simulink model "GNC2026"  (R2024b)
settings: Solver=ode4  StartTime=0.0  StopTime=tsim  FixedStep=baseRate
values from neighbouring files (symbols this model uses):
  a = 1    [Run_Initializer.m]    (also in UKFoptimization.m)
  a1 = 0.236940    (= 0.23694)    [DrawARM.m]    (also in Run_Initializer.m = 2)
  a2 = 0.281536    [DrawARM.m]    (also in Run_Initializer.m = 2)
  a3 = 0.0621    [DrawARM.m]    (also in Run_Initializer.m = 2)
  A_c = eye(3)    [Run_Initializer.m]
  alpha = diag([a1; a2; a3])    [Run_Initializer.m]    (also in overlapping_trajectories.m = alpha_values1(ii); plotTrajectory.m = alpha_values(ii); plotfig.m = alpha_values(ii))
  b = 2    [Run_Initializer.m]    (also in UKFoptimization.m)
  b0 = 0.230400    (= 0.2304)    [DrawARM.m]
  b1 = 0.078980    (= 0.07898)    [DrawARM.m]
  b2 = 0.070384    [DrawARM.m]
  b3 = 0.070685    [DrawARM.m]
  CVrate = 1/5    (= 0.2)    [Run_Initializer.m]
  dt = baseRate    [Run_Initializer.m]    (also in UKFoptimization.m = 0.05; rms_plots.m = median(diff(tA)))
  F_u = zeros(3,1)    [Run_Initializer.m]
  fNum = 1    [Run_Initializer.m]
  gamma = r - (excess + shrink + bracketwidth)    (= 0.05023)    [DrawSpacecraft.m]    (also in Run_Initializer.m = diag([g1; g2; g3]))
  Gamma1_el = 0.12    [Run_Initializer.m]
  Gamma1_sh = 0.005    [Run_Initializer.m]
  Gamma1_wr = 0.025    [Run_Initializer.m]
  Gamma2_el = 5    [Run_Initializer.m]
  Gamma2_sh = 5    [Run_Initializer.m]
  Gamma2_wr = 5    [Run_Initializer.m]
  Gamma3_el = 10    [Run_Initializer.m]
  Gamma3_sh = 40    [Run_Initializer.m]
  Gamma3_wr = 40    [Run_Initializer.m]
  Gamma4_el = 0.039    [Run_Initializer.m]
  Gamma4_sh = 0.015    [Run_Initializer.m]
  Gamma4_wr = 0.029    [Run_Initializer.m]
  Gamma5_el = 800    [Run_Initializer.m]
  Gamma5_sh = 800    [Run_Initializer.m]
  Gamma5_wr = 800    [Run_Initializer.m]
  Gamma6_el = 0.000001    (= 1e-06)    [Run_Initializer.m]
  Gamma6_sh = 0.005    [Run_Initializer.m]
  Gamma6_wr = 0.02    [Run_Initializer.m]
  k = 5    [Run_Initializer.m]    (also in UKFoptimization.m)
  Kd_elarm = 0.8    [Run_Initializer.m]
  Kd_sharm = 1.0    (= 1)    [Run_Initializer.m]
  Kd_wrarm = 0.6    [Run_Initializer.m]
  Kp_elarm = 1.2    [Run_Initializer.m]
  Kp_sharm = 1.5    [Run_Initializer.m]
  Kp_wrarm = 1.0    (= 1)    [Run_Initializer.m]
  Mc_inv = inv(M_c)    [Run_Initializer.m]
  Phi = 73.2749*pi/180    (= 1.27888826407)    [DrawARM.m]
  PWMFreq = 5    [Run_Initializer.m]
  R = [cos(theta) -sin(theta) ... (first row only)    [Run_Initializer.m]    (also in UKFoptimization.m = diag([rx, rx, rt]))
  sep1 = 0.60    (= 0.6)    [Run_Initializer.m]
  sep2 = 0.30    (= 0.3)    [Run_Initializer.m]
  sep3 = 0.30    (= 0.3)    [Run_Initializer.m]
  Tz_lim_elarm = .1    (= 0.1)    [Run_Initializer.m]
  Tz_lim_sharm = .1    (= 0.1)    [Run_Initializer.m]
  Tz_lim_wrarm = .1    (= 0.1)    [Run_Initializer.m]
  VISinLoop = 1    [Run_Initializer.m]
  X1_blk = 0.4    [Run_Initializer.m]
  X2_blk = 0.4    [Run_Initializer.m]
  X3_blk = 0.4    [Run_Initializer.m]
  Y1_blk = 0.4    [Run_Initializer.m]
  Y2_blk = 0.4    [Run_Initializer.m]
  Y3_blk = 0.4    [Run_Initializer.m]
undefined symbols (not defined in the file or in its folder): baseRate, dataRate, DiscIntNeverNeededParam, drop_states_ARM, drop_states_BLACK, drop_states_BLUE, drop_states_RED, F_red_X_nominal, F_red_Y_nominal, F_thrusters_BLACK, F_thrusters_BLUE, F_thrusters_RED, home_states_BLACK, home_states_BLUE, home_states_RED, IBLACK, IBLUE, IDIST, IEE, init_states_BLACK, init_states_BLUE, init_states_RED, IPROX, IRED, K_BLACK, K_BLUE, K_RED, Kd_tb, Kd_tblue, Kd_tr, Kd_xb, Kd_xblue, Kd_xr, Kd_yb, Kd_yblue, Kd_yr, Kp_tb, Kp_tblue, Kp_tr, Kp_xb, Kp_xblue, Kp_xr, Kp_yb, Kp_yblue, Kp_yr, mBLACK, mBLUE, mDIST, mEE, mPROX, mRED, Phase0_End, Phase1_End, Phase2_End, Phase3_End, Phase3_SubPhase1_End, Phase3_SubPhase2_End, Phase3_SubPhase3_End, Phase3_SubPhase4_End, Phase4_End ... (+10)
libraries: simulink x30, nvidiaSharedBlocks x20, MainLibrary x5, dspinverses x3, commrandsrc3 x1, nvidiaIMUSensorslib x1
(part 9 of 9)

== matlab function GNC2026/PhaseSpace Camera Code/Use Hardware to Obtain States/Store BLACK Data/Simulated Noise  (HARDWARE)/Artificial isValid Flag/MATLAB Function1 ==
  data: isValue output; baseRate parameter
function isValue = fcn(baseRate)

persistent k

if isempty(k)
    k = 0;
end

time = k*baseRate;

if time > 65
    isValue = 1;
else
    isValue = 0;
end

k = k+1;

end

== matlab function GNC2026/Navigation Filter/If Action Subsystem/EKF/EKF ==
  data: black_cv_pose input; pose output; velocity output; baseRate parameter; CVrate parameter; confidence output
% Ally Colla
% Chris El-Asmar
% MEKF DOT 2025 

function [pose, velocity, confidence] = MEKF(black_cv_pose, baseRate, CVrate)

persistent converge

if isempty(converge)
    converge = 0;
end

% Different sampling rate
% baseRate = 0.1;

% process noise covariance for propogation
Qx = 1e-8;
Qy = 1e-8;
Qtheta = 1e-8;

% measurement noise covariance for measurement update
Rx = 5e-3;
Ry = 5e-3; 
Rtheta = 5e-3; 
R = diag([Rx, Ry, Rtheta]); 

% filter initial conditions and memory 
persistent x P run theta theta_prev initial_theta
if isempty(run) % check if MEKF has run
    x = zeros(6,1); % x = state vector,(x,y,vx, vy, theta, omega)
    P = diag([1 1 0.05 0.05 1 0.05]); % initial uncertainties based off the spike magnitudes of +/- 1
    run = true;
    theta = 0; 
    theta_prev = 0;
    initial_theta = false;
end

% PROPOGATION

% setting up state transition matrix for 6 dof
phi = eye(6); 
phi(1,3) = baseRate; % updates x position, xnew = x + vx*dt
phi(2,4) = baseRate; % updates y position, ynew = y + vy*dt
phi(5,6) = baseRate; % updates theta position, thetanew = theta + w*dt

x = phi*x; % equation 16 in paper, Wk = 0

% setting up gamma matrix
% take bottom left of matrix in equation 17
% neglecting linear and angular accelerations
% planar rotation only, so no ap (attitude error)
gamma = zeros(6,3);  
gamma(3,1) = 1; % vx
gamma(4,2) = 1; % vy
gamma(6,3) = 1; % omega

Qc = diag([Qx, Qy, Qtheta]);
Qd = Qc*baseRate; % discrete covariance

% calculating covariance of state estimation error
P = phi*P*phi.' + gamma*Qd*gamma.'; 

% MEASUREMENT UPDATE AND OUTLIER REJECTION
yk = black_cv_pose(:); % measurement vector from equation 23

H = zeros(3,6);
H(1,1) = 1; % x
H(2,2) = 1; % y
H(3,5) = 1; % theta

% predicted measurement and innovation
ik = yk - H*x; % innovation equation, before equation 25
if norm(ik) < 0.05
    converge = 1;
end
confidence = converge;

% wrapping theta
wrap = atan2(sin(x(5)), cos(x(5))); % wrap theta from CV
ik(3) = atan2(sin(yk(3) - wrap), cos(yk(3) - wrap)); % wrap the difference

% innovation covariance
E_ik = H*P*H.' + R; % linearized approximation, equation 26 in paper 

% std deviation, expected uncertainty 
sxx = sqrt(max(E_ik(1,1), 1e-10)); % avoids zeros in calculation
syy = sqrt(max(E_ik(2,2), 1e-10));
stt = sqrt(max(E_ik(3,3), 1e-10));

% data falls within 3 std deviations of the mean
k = 3; 

% compare innovation to expected uncertainty 
% flag to see if values are outside 3x std deviation
% values for check become zero if exceeds 3x std dev. 
check_x = abs(ik(1)) <= k * sxx;
check_y = abs(ik(2)) <= k * syy;
check_theta = abs(ik(3)) <= k * stt;

% keep the x,y and theta values that are in the range of 3x std dev.
keep = [check_x; check_y; check_theta];
if any(keep)
    H_new = H(keep, :); % updates H with only the accepted pose
    ik_new = ik(keep); % updates innovation with only the accepted pose
    R_new = diag(diag(R(keep, keep))); % updates covariance matrix and diagonalizes with accepted pose
    Eik_new = H_new*P*H_new.' + R_new; % equation 26 with only accepted pose
    Ks = (P*H_new.')/Eik_new; % kalman gain equation
    x = x + Ks*ik_new; % update states based on kalman gain
    I = eye(6);
    % Joseph form 
    P  = (I - Ks*H_new)*P*(I - Ks*H_new).' + Ks*R_new*Ks.';
end

% keeping theta continuous
if ~initial_theta
    theta_prev = atan2(sin(x(5)), cos(x(5))); % wraps first angle
    theta = theta_prev;
    initial_theta = true;
else
    theta_new = atan2(sin(x(5)), cos(x(5))); 
    true_rotation = atan2(sin(theta_new - theta_prev), ...
                   cos(theta_new - theta_prev)); % wraps the difference for true physical rotation (no 360 jump)
    theta = theta + true_rotation; % previous theta + change in theta wrt time
    theta_prev = theta_new; % set previous theta to new theta to continue loop
end
x(5) = theta; % making theta continuous

% extract positions and velocities from state vector
pose = [x(1); x(2); x(5)];
velocity = [x(3); x(4); x(6)];

end
%%
function [flag] = measurement_flag(baseRate, CVrate)

persistent k
if isempty(k)
    k = 0;
end

flag = 0;

if mod(k,CVrate/baseRate) == 0      
    flag = 1;     % new measurement available
end

k = k + 1;

end

== matlab function GNC2026/Thruster Control Code/Change BLACK Behavior/Rotate Forces to Body/Create Rotation Matrix ==
  data: Rz input; C_bI output
function C_bI = RotateFrame(Rz)

C_bI = [  cos(Rz) sin(Rz)
         -sin(Rz) cos(Rz) ];

end

== matlab function GNC2026/Navigation Filter/If Action Subsystem/UKF/Unscented Kalman Filter ==
  data: x_pre input; x_est output; confidence output; y input; isValid input; P_pre input; P_est output; dt parameter; b parameter; k parameter; a parameter; R parameter; baseRate parameter; CVrate parameter
% Nimish Dhawan
% Sukriti Kumar
% 2025

%%%%%%%%%%%%%%%%%%%%%%%%%%%%%%%%%%%%%%%%%%%%%%%%%%%%%%%%%%%%%%%%%%%%%%%%%
% Inputs
%%%%%%%%%%%%%%%%%%%%%%%%%%%%%%%%%%%%%%%%%%%%%%%%%%%%%%%%%%%%%%%%%%%%%%%%%
% x (6x1)   : state variable [x; y; theta; x_dot; y_dot; theta_dot] 
% X         : Sigma Points
% a, k, b   : unscented transform parameters
% lambda    : scaling parameter
% P (6x6)   : covarience matrix
% S (6x6)   : cholesky decomposition of P

%%%%%%%%%%%%%%%%%%%%%%%%%%%%%%%%%%%%%%%%%%%%%%%%%%%%%%%%%%%%%%%%%%%%%%%%%
% Output
%%%%%%%%%%%%%%%%%%%%%%%%%%%%%%%%%%%%%%%%%%%%%%%%%%%%%%%%%%%%%%%%%%%%%%%%%
% x_est
% P_est

function [x_est, confidence, P_est] = UKF(x_pre, y, isValid, P_pre, dt, b, k, a, R, ...
                                         baseRate, CVrate)

persistent converge

if isempty(converge)
    converge = 0;
end

n = 6;
lambda = a^2 * (n + k) - n;

% Allocating memory
wi_m    = zeros((2*n+1),1);
wi_c    = zeros((2*n+1),1);

% Rotation matrix to go from inertial to relative pose
C3 = eye(3);

% mean and covariance weights (Eq. 4.17f)
for i = 1 : (2*n+1)
    if i == 1
        wi_m(i) = lambda / (n+lambda);
        wi_c(i) = wi_m(i) + 1 - a^2 + b;
    else
        wi_m(i) = 1 / (2 * (n+lambda));
        wi_c(i) = wi_m(i);
    end
end

dynamics = @(x, dt) x + dt * [x(4:6); zeros(3,1)];

% Allocating memory
P_minus = zeros(n,n);
Xi_pre  = zeros(n,(2*n+1));
Fi      = zeros(n,(2*n+1));
x_minus = zeros(n,1);

S_pre = chol(P_pre)';    % Gives lower triangle
Q = 1e-10*eye(n);

% Sigma points calculation 
for i = 1:2*n+1 
    if i == 1
        Xi_pre(:,i) = x_pre;
    elseif i > 1 && i <= n+1
        Xi_pre(:,i) = x_pre + sqrt(n + lambda) * S_pre(:,i-1);
    else
        Xi_pre(:,i) = x_pre - sqrt(n + lambda) * S_pre(:,i-n-1);
    end
end

% Sigma points propagation 
for i = 1 : (2*n+1)
    u = Xi_pre(:,i);
    Fi(:,i) = dynamics(u, dt);
end

% Priori state estimate 
for i = 1 : (2*n+1)
    x_minus = x_minus + wi_m(i) * Fi(:,i);
end

% Priori covariance estimate 
for i = 1 : (2*n+1)
    Pi = wi_c(i) * (Fi(:,i) - x_minus) * (Fi(:,i) - x_minus)' + Q;
    P_minus = P_minus + Pi;
end


% =========================================================================
% CORRECTION
% =========================================================================
Xi_minus = zeros(n,(2*n+1));
h = zeros(3,(2*n+1));    
y_hat = zeros(3,1);     
P_xy = zeros(n,3);
P_yy = zeros(3,3);

S_minus = chol(P_minus)';        % Gives lower triangle

% Sigma points calculation 
for i = 1:2*n+1 
    if i == 1
        Xi_minus(:,i) = x_minus;
    elseif i > 1 && i <= n+1
        Xi_minus(:,i) = x_minus + sqrt(n + lambda) * S_minus(:,i-1);
    else
        Xi_minus(:,i) = x_minus - sqrt(n + lambda) * S_minus(:,i-n-1);
    end
end

% Estimated measurement calculation 
for i = 1 : (2*n+1)
    h(:,i) = C3*Xi_minus(1:3,i);
    y_hat = y_hat + wi_m(i) * h(:,i);
end

% Residual
r = y - y_hat;
if norm(r) < 0.05 % 0.05 works, DO NOT CHANGE (experimentally validated)
    converge = 1;
end
confidence = converge;

% Estimated covariance calculation
for i = 1 : (2*n+1)
    P_yy = P_yy + wi_c(i) * (h(:,i)-y_hat) * (h(:,i)-y_hat)' + R;
    P_xy = P_xy + wi_c(i) * (Xi_minus(:,i) - x_minus) * (h(:,i)-y_hat)';
end

% Posteriori state estimate and covariance 
K = P_xy * inv(P_yy);

P_plus = P_minus - K * P_yy * K';
x_plus = x_minus + K * r;

% Mahalanobis distance

dM          = sqrt(r' * inv(P_yy) * r);
isOutlier   = dM > chi2inv(0.997, 3);

if isOutlier == 1
    P_plus = P_minus;
    x_plus = x_minus;
end

newMeas= measurement_flag(baseRate, CVrate);

if isValid == 1 && newMeas == 1 
    x_est = x_plus;
    P_est = P_plus;
else
    x_est = x_minus;
    P_est = P_minus;
end

end

%%
function [flag] = measurement_flag(baseRate, CVrate)

persistent k
if isempty(k)
    k = 0;
end

flag = 0;

if mod(k,CVrate/baseRate) == 0      
    flag = 1;     % new measurement available
end

k = k + 1;

end

== matlab function GNC2026/Thruster Control Code/Change BLUE Behavior/Calculate Duty Cycle/Generate Initial Guess/MATLAB Function ==
  data: H output; thruster_dist2CG_BLUE parameter; F_thrusters_BLUE parameter
function H = MakeH(thruster_dist2CG_BLUE,F_thrusters_BLUE)

    Vec1 = [ -1
             -1
              0 
              0
              1
              1
              0
              0 ];
          
    Vec2 = [  0
              0
              1
              1
              0
              0
             -1
             -1 ];
         
    Vec3 = thruster_dist2CG_BLUE./1000;
    
    Mat1 = [Vec1, Vec2, Vec3]';
    
    Mat2 = diag((F_thrusters_BLUE./2));
    
    H    = Mat1*Mat2;

end

== matlab function GNC2026/Navigation Filter/If Action Subsystem/EKF/Camera to Inertial Frame ==
  data: r_C_I input; r_T_I output; r_REL_C input
function r_T_I  = CIB(r_C_I, r_REL_C)
l_cam_x    = 0.125; %m, offset in x from origin of Red, left camera
l_cam_y    = 0.03; %m, offset in y from origin of Red, left camera
LAR_x      = 0.145; %m

r_REL_C(1:2) = r_REL_C(1:2) + [l_cam_x; l_cam_y];
th_C         = r_C_I(3);
th_REL       = r_REL_C(3);
th_T         = th_C+th_REL;

C_IC         = [cos(th_C) -sin(th_C); sin(th_C) cos(th_C)]; % Chaser to inertial ref frame rotation matrix
C_IT         = [cos(th_T) -sin(th_T); sin(th_T) cos(th_T)]; % Target to inertial ref frame rotation matrix
xy_T_I       = r_C_I(1:2) + C_IC*r_REL_C(1:2);

r_T_I        = [xy_T_I-C_IT*[LAR_x;0]; th_T];
end

== matlab function GNC2026/Thruster Control Code/Change BLUE Behavior/Calculate Duty Cycle/Rotate Forces to Inertial/Create Rotation Matrix ==
  data: Rz input; C_Ib output
function C_Ib = RotateFrame(Rz)

C_bI = [  cos(Rz) sin(Rz)
         -sin(Rz) cos(Rz) ];

C_Ib = inv(C_bI);

end

== matlab function GNC2026/Simulate Plant Dynamics/BLACK Dynamics/Simulated Noise /Inertial to Camera Frame (SOFTWARE) ==
  data: r_C input; r_REL output; r_T input
% Rotation matrix to go from inertial to relative
function r_REL = CBI(r_C, r_T)
l_cam_x    = 0.125; %m, offset in x from origin of Red, left camera
l_cam_y    = 0.03; %m, offset in y from origin of Red, left camera
th_C       = r_C(3);
th_T       = r_T(3);
d_xy       = r_T(1:2) - r_C(1:2);
C_CI       = [cos(th_C) sin(th_C); -sin(th_C) cos(th_C)]; % Chaser to inertial ref frame rotation matrix
r_REL      = [C_CI*d_xy; th_T - th_C];
r_REL(1:2) = r_REL(1:2) - [l_cam_x; l_cam_y];
end

== matlab function GNC2026/Thruster Control Code/Change BLUE Behavior/Rotate Forces to Body/Create Rotation Matrix ==
  data: Rz input; C_bI output
function C_bI = RotateFrame(Rz)

C_bI = [  cos(Rz) sin(Rz)
         -sin(Rz) cos(Rz) ];

end

== matlab function GNC2026/Thruster Control Code/Change RED Behavior/Calculate Duty Cycle/Generate Initial Guess/MATLAB Function ==
  data: H output; thruster_dist2CG_RED parameter; F_thrusters_RED parameter
function H = MakeH(thruster_dist2CG_RED,F_thrusters_RED)

    Vec1 = [ -1
             -1
              0 
              0
              1
              1
              0
              0 ];
          
    Vec2 = [  0
              0
              1
              1
              0
              0
             -1
             -1 ];
         
    Vec3 = thruster_dist2CG_RED./1000;
    
    Mat1 = [Vec1, Vec2, Vec3]';
    
    Mat2 = diag((F_thrusters_RED./2));
    
    H    = Mat1*Mat2;

end

== matlab function GNC2026/Thruster Control Code/Change RED Behavior/Calculate Duty Cycle/MATLAB Function5 ==
  data: H_final output; u_desired input; duty_cycles output; x0 input; thruster_dist2CG_RED parameter; F_red_X_nominal parameter; F_red_Y_nominal parameter; max_iters parameter; tol parameter
function [H_final, duty_cycles] = optimize_duty_cycle_with_decay( ...
    u_desired, x0, thruster_dist2CG_RED, F_red_X_nominal, F_red_Y_nominal, max_iters, tol)
    %OPTIMIZE_DUTY_CYCLE_WITH_DECAY 
    %   Iteratively optimizes thruster duty cycles while updating thrust decay.
    %
    %   Inputs:
    %       u_desired           - Desired force/torque vector [Fx; Fy; M] (3x1)
    %       x0                  - Initial guess for duty cycles (8x1)
    %       thruster_dist2CG_RED- Distances of thrusters from CG (vector, mm)
    %       F_red_X_nominal     - Nominal X-direction thruster force (scalar, N)
    %       F_red_Y_nominal     - Nominal Y-direction thruster force (scalar, N)
    %       max_iters           - Maximum optimization iterations
    %       tol                 - Convergence tolerance (on duty cycles)
    %
    %   Outputs:
    %       H_final     - Final H-matrix including thrust decay (3x8)
    %       duty_cycles - Optimized duty cycles (8x1)
    %

    % ---------------------------
    % Initialization
    % ---------------------------
    num_thrusters      = length(x0); %#ok<NASGU> % reserved if needed later
    duty_cycles        = x0;                     % current solution
    thrust_decay_factor = 1;                     % initial decay
    prev_duty_cycles   = duty_cycles + 2*tol;    % force first iteration

    % ---------------------------
    % Iterative optimization
    % ---------------------------
    for iter = 1:max_iters
        % Build system matrix H with current decay factor
        H = MakeHWithDecay(thruster_dist2CG_RED, F_red_X_nominal, ...
                           thrust_decay_factor, F_red_Y_nominal);

        % Solve constrained least squares (box constraints: 0 ≤ x ≤ 1)
        duty_cycles = custom_constrained_least_squares(H, u_desired, duty_cycles);

        % Update decay factor based on the current duty cycles
        [thrust_decay_factor, ~] = check_thrust_decay(duty_cycles);

        % Check convergence (∞-norm difference)
        if norm(duty_cycles - prev_duty_cycles, Inf) < tol
            H_final = MakeHWithDecayRecalculateForce(thruster_dist2CG_RED, ...
                        F_red_X_nominal, thrust_decay_factor, F_red_Y_nominal);
            return;
        end

        % Update reference for next iteration
        prev_duty_cycles = duty_cycles;
    end

    % If not converged within max_iters, return final H with last decay
    H_final = MakeHWithDecayRecalculateForce(thruster_dist2CG_RED, ...
                F_red_X_nominal, thrust_decay_factor, F_red_Y_nominal);
end


% ========================================================================
% Custom Constrained Least Squares Solver
% ========================================================================
function x_opt = custom_constrained_least_squares(H, b, x0)
    %CUSTOM_CONSTRAINED_LEAST_SQUARES
    %   Solves min_x ||H*x - b||^2 subject to 0 <= x <= 1
    %   using projected gradient descent with backtracking line search.
    %
    %   Inputs:
    %       H   - System matrix (3x8)
    %       b   - Desired vector (3x1)
    %       x0  - Initial guess (8x1)
    %
    %   Output:
    %       x_opt - Optimal duty cycle vector (8x1)

    % Parameters
    max_iterations = 100;
    tolerance      = 1e-6;
    alpha          = 0.01;  % initial step size
    beta           = 0.5;   % backtracking factor

    % Initialization
    x      = x0;
    x_prev = x0 + 2*tolerance;

    % Precompute matrices
    HtH = H' * H;
    Htb = H' * b;

    for iter = 1:max_iterations
        % Gradient of ||H*x - b||^2
        gradient = 2 * (HtH*x - Htb);

        % Store objective for comparison
        current_obj = norm(H*x - b)^2;

        % Backtracking line search
        step_size = alpha;
        for ls_iter = 1:20
            x_new = x - step_size * gradient;
            x_new = max(0, min(1, x_new)); % project into [0,1]

            new_obj = norm(H*x_new - b)^2;
            if new_obj < current_obj
                break; % accept step
            else
                step_size = step_size * beta;
            end
        end

        % Update
        x = x_new;

        % Convergence check
        if norm(x - x_prev) < tolerance
            break;
        end

        % Adaptive step size tuning
        if iter > 1 && new_obj < current_obj
            alpha = min(alpha * 1.1, 0.1); % speed up if progress
        else
            alpha = alpha * 0.9;           % slow down otherwise
        end

        % Store for next iteration
        x_prev = x;
    end

    x_opt = x;
end


% ========================================================================
% Construct H-matrix (with decay factor)
% ========================================================================
function H = MakeHWithDecay(thruster_dist2CG, F_X_nominal, thrust_decay_factor, F_Y_nominal)
    %MAKEHWITHDECAY
    %   Builds the H matrix that maps thruster duty cycles to [Fx; Fy; M],
    %   applying thrust decay.
    %
    %   Outputs H as (3x8)

    % Convert thruster arm distances to meters
    adjusted_dist = thruster_dist2CG / 1000;

    % Thruster directions (X, Y, and moment arm)
    Vec1 = [-1; -1;  0;  0;  1;  1;  0;  0]; % X
    Vec2 = [ 0;  0;  1;  1;  0;  0; -1; -1]; % Y
    Vec3 = adjusted_dist;                    % moment (Z)

    Mat1 = [Vec1, Vec2, Vec3]';

    % Thruster forces (scaled by decay)
    F_thrusters = [F_X_nominal; F_X_nominal; ...
                   F_Y_nominal; F_Y_nominal; ...
                   F_X_nominal; F_X_nominal; ...
                   F_Y_nominal; F_Y_nominal] * thrust_decay_factor;

    % Build diagonal scaling
    Mat2 = diag(F_thrusters / 2);

    % Final mapping
    H = Mat1 * Mat2;
end


% ========================================================================
% Construct H-matrix (recalculate full force with decay)
% ========================================================================
function H = MakeHWithDecayRecalculateForce(thruster_dist2CG, F_X_nominal, thrust_decay_factor, F_Y_nominal)
    %MAKEHWITHDECAYRECALCULATEFORCE
    %   Same as MakeHWithDecay but applies full nominal force scaling.

    adjusted_dist = thruster_dist2CG / 1000;

    Vec1 = [-1; -1;  0;  0;  1;  1;  0;  0];
    Vec2 = [ 0;  0;  1;  1;  0;  0; -1; -1];
    Vec3 = adjusted_dist;

    Mat1 = [Vec1, Vec2, Vec3]';

    F_thrusters = [F_X_nominal; F_X_nominal; ...
                   F_Y_nominal; F_Y_nominal; ...
                   F_X_nominal; F_X_nominal; ...
                   F_Y_nominal; F_Y_nominal] * thrust_decay_factor;

    Mat2 = diag(F_thrusters);

    H = Mat1 * Mat2;
end


% ========================================================================
% Thrust Decay Update Rule
% ========================================================================
function [thrust_decay_factor, count] = check_thrust_decay(PWMs)
    %CHECK_THRUST_DECAY
    %   Updates thrust decay factor based on average duty cycle.
    %
    %   Inputs:
    %       PWMs - Duty cycle vector (8x1)
    %
    %   Outputs:
    %       thrust_decay_factor - Adjusted decay factor (scalar)
    %       count               - Number of active thrusters

    % Normalize if needed
    if max(PWMs) > 1
        PWMs = PWMs / max(PWMs);
    end
    
    % Active thrusters
    count = sum(PWMs > 0);
    
    % Mean duty cycle (only active thrusters)
    avg_duty = sum(max(PWMs, 0)) / max(count, 1);
    
    % Update rule (piecewise)
    if avg_duty < 0.3 || count == 0
        thrust_decay_factor = 1;
    else
        thrust_decay_factor = max(0.6 - 2*avg_duty + 1, 0.5);
    end
end

== matlab function GNC2026/Thruster Control Code/Change BLUE Behavior/Calculate Duty Cycle/MATLAB Function1 ==
  data: ThrustPer_Final output; ThrustPer input; PWMFreq parameter
function ThrustPer_Final  = ThrusterSat(ThrustPer, PWMFreq)

    ValveTime       = 0.007;
    TControl        = 1/PWMFreq;

    ThrustPer_Final = zeros(8,1);
    
    if max(ThrustPer) > 1
        ThrustPer_Sat = ThrustPer/max(ThrustPer);
    else
        ThrustPer_Sat = ThrustPer;
    end
    
    for i = 1:8
        if ThrustPer_Sat(i) > ValveTime/TControl 
            ThrustPer_Final(i) = ThrustPer_Sat(i);
        else
            ThrustPer_Final(i) = 0;
        end
    end


end

== matlab function GNC2026/Navigation Filter/If Action Subsystem/UKF/Camera to Inertial Frame ==
  data: r_C_I input; r_T_I output; r_REL_C input
function r_T_I  = CIB(r_C_I, r_REL_C)
l_cam_x    = 0.125; %m, offset in x from origin of Red, left camera
l_cam_y    = 0.03;  %m, offset in y from origin of Red, left camera
LAR_x      = 0.145; %m

r_REL_C(1:2) = r_REL_C(1:2) + [l_cam_x; l_cam_y];
th_C         = r_C_I(3);
th_REL       = r_REL_C(3);
th_T         = th_C+th_REL;

C_IC         = [cos(th_C) -sin(th_C); sin(th_C) cos(th_C)]; % Chaser to inertial ref frame rotation matrix
C_IT         = [cos(th_T) -sin(th_T); sin(th_T) cos(th_T)]; % Target to inertial ref frame rotation matrix
xy_T_I       = r_C_I(1:2) + C_IC*r_REL_C(1:2);

r_T_I        = [xy_T_I-C_IT*[LAR_x;0]; th_T];
end

== matlab function GNC2026/Simulate Plant Dynamics/BLACK Dynamics/Simulated Noise /Unwrap/Unwrap/MATLAB Function ==
  data: u input; y output; u_pre input; y_pre input; u_next output
function [y, u_next] = fcn(u, u_pre, y_pre)

% Nimish Dhawan 2025
% Carleton University

%%%%%%%%%%%%%%%%%%%%%%%%%%%%%%%%%%%%%%%%%%%%%%%%%%%%%%%%%%%%%%%%%%%%%%%%%
% Inputs
%%%%%%%%%%%%%%%%%%%%%%%%%%%%%%%%%%%%%%%%%%%%%%%%%%%%%%%%%%%%%%%%%%%%%%%%%
% u (rad)       : current wrapped angle
% u_pre (rad)   : previous wrapped angle
% y_pre (rad)   : previous unwrapped angle

%%%%%%%%%%%%%%%%%%%%%%%%%%%%%%%%%%%%%%%%%%%%%%%%%%%%%%%%%%%%%%%%%%%%%%%%%
% Output
%%%%%%%%%%%%%%%%%%%%%%%%%%%%%%%%%%%%%%%%%%%%%%%%%%%%%%%%%%%%%%%%%%%%%%%%%
% y (rad)       : unwrapped angle
% u_next (rad)  : next wrapped angle

x = mod((u-u_pre)+pi, 2*pi) - pi;

y = y_pre + x;
u_next = u;

end

== matlab function GNC2026/Thruster Control Code/Change RED Behavior/Calculate Duty Cycle/Rotate Forces to Inertial/Create Rotation Matrix ==
  data: Rz input; C_Ib output
function C_Ib = RotateFrame(Rz)

C_bI = [  cos(Rz) sin(Rz)
         -sin(Rz) cos(Rz) ];

C_Ib = inv(C_bI);

end

== matlab function GNC2026/Thruster Control Code/Change RED Behavior/Rotate Forces to Body/Create Rotation Matrix ==
  data: Rz input; C_bI output
function C_bI = RotateFrame(Rz)

C_bI = [  cos(Rz) sin(Rz)
         -sin(Rz) cos(Rz) ];

end

== matlab function GNC2026/Simulate Plant Dynamics/BLACK Dynamics/Simulated Noise /Unwrap/Unwrap1/MATLAB Function ==
  data: u input; y output; y_pre input; init_states_BLACK parameter
function y  = fcn(u, y_pre, init_states_BLACK)

% Nimish Dhawan 2025
% Carleton University

persistent hold

if isempty(hold)
    hold = init_states_BLACK(3);
end

%%%%%%%%%%%%%%%%%%%%%%%%%%%%%%%%%%%%%%%%%%%%%%%%%%%%%%%%%%%%%%%%%%%%%%%%%
% Inputs
%%%%%%%%%%%%%%%%%%%%%%%%%%%%%%%%%%%%%%%%%%%%%%%%%%%%%%%%%%%%%%%%%%%%%%%%%
% u (rad)       : current wrapped angle
% u_pre (rad)   : previous wrapped angle
% y_pre (rad)   : previous unwrapped angle

%%%%%%%%%%%%%%%%%%%%%%%%%%%%%%%%%%%%%%%%%%%%%%%%%%%%%%%%%%%%%%%%%%%%%%%%%
% Output
%%%%%%%%%%%%%%%%%%%%%%%%%%%%%%%%%%%%%%%%%%%%%%%%%%%%%%%%%%%%%%%%%%%%%%%%%
% y (rad)       : unwrapped angle
% u_next (rad)  : next wrapped angle

x = mod((u-hold)+pi, 2*pi) - pi;

y = y_pre + x;
hold = u;

end

== matlab function GNC2026/Navigation Filter/If Action Subsystem/UKF/Unwrap/Unwrap/MATLAB Function ==
  data: u input; y output; u_pre input; y_pre input; u_next output
function [y, u_next] = fcn(u, u_pre, y_pre)

% Nimish Dhawan 2025
% Carleton University

%%%%%%%%%%%%%%%%%%%%%%%%%%%%%%%%%%%%%%%%%%%%%%%%%%%%%%%%%%%%%%%%%%%%%%%%%
% Inputs
%%%%%%%%%%%%%%%%%%%%%%%%%%%%%%%%%%%%%%%%%%%%%%%%%%%%%%%%%%%%%%%%%%%%%%%%%
% u (rad)       : current wrapped angle
% u_pre (rad)   : previous wrapped angle
% y_pre (rad)   : previous unwrapped angle

%%%%%%%%%%%%%%%%%%%%%%%%%%%%%%%%%%%%%%%%%%%%%%%%%%%%%%%%%%%%%%%%%%%%%%%%%
% Output
%%%%%%%%%%%%%%%%%%%%%%%%%%%%%%%%%%%%%%%%%%%%%%%%%%%%%%%%%%%%%%%%%%%%%%%%%
% y (rad)       : unwrapped angle
% u_next (rad)  : next wrapped angle

x = mod((u-u_pre)+pi, 2*pi) - pi;

y = y_pre + x;
u_next = u;

end

== matlab function GNC2026/Navigation Filter/If Action Subsystem/UKF/Unwrap/Unwrap1/MATLAB Function ==
  data: u input; y output; y_pre input; init_states_BLACK parameter
function y  = fcn(u, y_pre, init_states_BLACK)

% Nimish Dhawan 2025
% Carleton University

persistent hold

if isempty(hold)
    hold = init_states_BLACK(3);
end

%%%%%%%%%%%%%%%%%%%%%%%%%%%%%%%%%%%%%%%%%%%%%%%%%%%%%%%%%%%%%%%%%%%%%%%%%
% Inputs
%%%%%%%%%%%%%%%%%%%%%%%%%%%%%%%%%%%%%%%%%%%%%%%%%%%%%%%%%%%%%%%%%%%%%%%%%
% u (rad)       : current wrapped angle
% u_pre (rad)   : previous wrapped angle
% y_pre (rad)   : previous unwrapped angle

%%%%%%%%%%%%%%%%%%%%%%%%%%%%%%%%%%%%%%%%%%%%%%%%%%%%%%%%%%%%%%%%%%%%%%%%%
% Output
%%%%%%%%%%%%%%%%%%%%%%%%%%%%%%%%%%%%%%%%%%%%%%%%%%%%%%%%%%%%%%%%%%%%%%%%%
% y (rad)       : unwrapped angle
% u_next (rad)  : next wrapped angle

x = mod((u-hold)+pi, 2*pi) - pi;

y = y_pre + x;
hold = u;

end

== matlab function GNC2026/Thruster Control Code/Change BLACK Behavior/Calculate Duty Cycle/MATLAB Function1 ==
  data: ThrustPer_Final output; ThrustPer input; PWMFreq parameter
function ThrustPer_Final  = ThrusterSat(ThrustPer, PWMFreq)

    ValveTime       = 0.007;
    TControl        = 1/PWMFreq;

    ThrustPer_Final = zeros(8,1);
    
    if max(ThrustPer) > 1
        ThrustPer_Sat = ThrustPer/max(ThrustPer);
    else
        ThrustPer_Sat = ThrustPer;
    end
    
    for i = 1:8
        if ThrustPer_Sat(i) > ValveTime/TControl 
            ThrustPer_Final(i) = ThrustPer_Sat(i);
        else
            ThrustPer_Final(i) = 0;
        end
    end


end

== matlab function GNC2026/PhaseSpace Camera Code/Use Hardware to Obtain States/Store BLACK Data/Simulated Noise  (HARDWARE)/Sample and Hold ==
  data: y output; u input; CVrate parameter; baseRate parameter
function y  = fcn(u, CVrate, baseRate)
% Description:
% Sampling and holding values
% Input: 
% u [3x1]: CV Data
% Output:
% y [3x1]: Sampled Data

persistent k y_hold

% Initialize 
if isempty(k)
    k = 0;
    y_hold = u;
end

% Sample the value at every second step
if mod(k,CVrate/baseRate) == 0
    y_hold = u;   
end

y = y_hold;

k = k+1;

end

== matlab function GNC2026/3 - Control/Default LQR Control (RED)/Calculate Error/MATLAB Function ==
  data: Rz_path input; Rz_error output; Rz_measured input
function Rz_error = SmoothAngularDifference(Rz_path, Rz_measured)

    Rz_error = mod(Rz_measured-Rz_path+pi, 2*pi)-pi;


end

== matlab function GNC2026/PhaseSpace Camera Code/Use Hardware to Obtain States/Store BLACK Data/Simulated Noise  (HARDWARE)/Unwrap/Unwrap/MATLAB Function ==
  data: u input; y output; u_pre input; y_pre input; u_next output
function [y, u_next] = fcn(u, u_pre, y_pre)

% Nimish Dhawan 2025
% Carleton University

%%%%%%%%%%%%%%%%%%%%%%%%%%%%%%%%%%%%%%%%%%%%%%%%%%%%%%%%%%%%%%%%%%%%%%%%%
% Inputs
%%%%%%%%%%%%%%%%%%%%%%%%%%%%%%%%%%%%%%%%%%%%%%%%%%%%%%%%%%%%%%%%%%%%%%%%%
% u (rad)       : current wrapped angle
% u_pre (rad)   : previous wrapped angle
% y_pre (rad)   : previous unwrapped angle

%%%%%%%%%%%%%%%%%%%%%%%%%%%%%%%%%%%%%%%%%%%%%%%%%%%%%%%%%%%%%%%%%%%%%%%%%
% Output
%%%%%%%%%%%%%%%%%%%%%%%%%%%%%%%%%%%%%%%%%%%%%%%%%%%%%%%%%%%%%%%%%%%%%%%%%
% y (rad)       : unwrapped angle
% u_next (rad)  : next wrapped angle

x = mod((u-u_pre)+pi, 2*pi) - pi;

y = y_pre + x;
u_next = u;

end

== matlab function GNC2026/Simulate Plant Dynamics/BLACK Dynamics/Simulated Noise /Sample and Hold ==
  data: y output; u input; CVrate parameter; baseRate parameter
function y  = fcn(u, CVrate, baseRate)
% Description:
% Sampling and holding values
% Input: 
% u [3x1]: CV Data
% Output:
% y [3x1]: Sampled Data

persistent k y_hold

% Initialize 
if isempty(k)
    k = 0;
    y_hold = u;
end

% Sample the value at every second step
if mod(k,CVrate/baseRate) == 0
    y_hold = u;   
end

y = y_hold;

k = k+1;

end

== matlab function GNC2026/Simulate Plant Dynamics/BLACK Dynamics/Simulated Noise /MATLAB Function1 ==
  data: data output; LARstates_C_B input; isValid output; baseRate parameter
function [data, isValid] = fcn(LARstates_C_B, baseRate)

persistent k

if isempty(k)
    k = 0;
end

time = k*baseRate;

% Extracting LAR states
x = LARstates_C_B(1);
y = LARstates_C_B(2);

% Angle between normal and LOS vector
lambda = atand(y/x);

% Send isValue = 0 when target LAR is out of FOV
% if abs(lambda) > 40
%     isValid = 0;
% else
%     isValid = 1;
% end
isValid = 1;

k = k+1;

if isValid == 1
    data = [0;0;0];
else
    data = LARstates_C_B;
end

% data = LARstates_C_B;
% isValid = 1;

end

== matlab function GNC2026/2 - Guidance/Custom PPL (RED)/End Effector Desired ==
  data: r_C input; r_T_I input; EEdesired output; thRel output; LOS_angle output
function [EEdesired, thRel, LOS_angle] = fcn(r_C, r_T_I)

LARstates_I = r_T_I;

LAR_x = 0.145; % LAR offset in target BoF, m
th_T  = r_T_I(3);
C_IT  = [cos(th_T) -sin(th_T); sin(th_T) cos(th_T)]; % Target to inertial ref frame rotation matrix

LARstates_I(1:2) = r_T_I(1:2) + C_IT*[LAR_x;0];
LARstates_REL = CBI(r_C, LARstates_I);

EEdesired = LARstates_REL + [0.02; 0.15; 0];
thRel     = LARstates_REL(3);
LOS_angle = atan(LARstates_REL(2)/LARstates_REL(1));

end
%%
% Rotation matrix to go from inertial to relative
function r_REL = CBI(r_C, r_T)
th_C       = r_C(3);
th_T       = r_T(3);
d_xy       = r_T(1:2) - r_C(1:2);
C_CI       = [cos(th_C) sin(th_C); -sin(th_C) cos(th_C)]; % Chaser to inertial ref frame rotation matrix
r_REL      = [C_CI*d_xy; th_T - th_C];
r_REL(1:2) = r_REL(1:2);
end

== matlab function GNC2026/Simulate Plant Dynamics/BLACK Dynamics/Simulated Noise /BLK CoM to LAR ==
  data: r_T_I input; LARstates_I output
% Calculates position vector of LAR based on position vector of Target CoM 
function LARstates_I = fcn(r_T_I)

LARstates_I = r_T_I;

LAR_x = 0.145; % LAR offset in target BoF, m
th_T  = r_T_I(3);
C_IT  = [cos(th_T) -sin(th_T); sin(th_T) cos(th_T)]; % Target to inertial ref frame rotation matrix


LARstates_I(1:2) = r_T_I(1:2) + C_IT*[LAR_x;0];

end

== matlab function GNC2026/PhaseSpace Camera Code/Use Hardware to Obtain States/Store BLACK Data/Simulated Noise  (HARDWARE)/Unwrap/Unwrap1/MATLAB Function ==
  data: u input; y output; y_pre input; init_states_BLACK parameter
function y  = fcn(u, y_pre, init_states_BLACK)

% Nimish Dhawan 2025
% Carleton University

persistent hold

if isempty(hold)
    hold = init_states_BLACK(3);
end

%%%%%%%%%%%%%%%%%%%%%%%%%%%%%%%%%%%%%%%%%%%%%%%%%%%%%%%%%%%%%%%%%%%%%%%%%
% Inputs
%%%%%%%%%%%%%%%%%%%%%%%%%%%%%%%%%%%%%%%%%%%%%%%%%%%%%%%%%%%%%%%%%%%%%%%%%
% u (rad)       : current wrapped angle
% u_pre (rad)   : previous wrapped angle
% y_pre (rad)   : previous unwrapped angle

%%%%%%%%%%%%%%%%%%%%%%%%%%%%%%%%%%%%%%%%%%%%%%%%%%%%%%%%%%%%%%%%%%%%%%%%%
% Output
%%%%%%%%%%%%%%%%%%%%%%%%%%%%%%%%%%%%%%%%%%%%%%%%%%%%%%%%%%%%%%%%%%%%%%%%%
% y (rad)       : unwrapped angle
% u_next (rad)  : next wrapped angle

x = mod((u-hold)+pi, 2*pi) - pi;

y = y_pre + x;
hold = u;

end

== matlab function GNC2026/Navigation Filter/If Action Subsystem/EKF/Unwrap/Unwrap/MATLAB Function ==
  data: u input; y output; u_pre input; y_pre input; u_next output
function [y, u_next] = fcn(u, u_pre, y_pre)

% Nimish Dhawan 2025
% Carleton University

%%%%%%%%%%%%%%%%%%%%%%%%%%%%%%%%%%%%%%%%%%%%%%%%%%%%%%%%%%%%%%%%%%%%%%%%%
% Inputs
%%%%%%%%%%%%%%%%%%%%%%%%%%%%%%%%%%%%%%%%%%%%%%%%%%%%%%%%%%%%%%%%%%%%%%%%%
% u (rad)       : current wrapped angle
% u_pre (rad)   : previous wrapped angle
% y_pre (rad)   : previous unwrapped angle

%%%%%%%%%%%%%%%%%%%%%%%%%%%%%%%%%%%%%%%%%%%%%%%%%%%%%%%%%%%%%%%%%%%%%%%%%
% Output
%%%%%%%%%%%%%%%%%%%%%%%%%%%%%%%%%%%%%%%%%%%%%%%%%%%%%%%%%%%%%%%%%%%%%%%%%
% y (rad)       : unwrapped angle
% u_next (rad)  : next wrapped angle

x = mod((u-u_pre)+pi, 2*pi) - pi;

y = y_pre + x;
u_next = u;

end

== matlab function GNC2026/Navigation Filter/If Action Subsystem/EKF/Unwrap/Unwrap1/MATLAB Function ==
  data: u input; y output; y_pre input; init_states_BLACK parameter
function y  = fcn(u, y_pre, init_states_BLACK)

% Nimish Dhawan 2025
% Carleton University

persistent hold

if isempty(hold)
    hold = init_states_BLACK(3);
end

%%%%%%%%%%%%%%%%%%%%%%%%%%%%%%%%%%%%%%%%%%%%%%%%%%%%%%%%%%%%%%%%%%%%%%%%%
% Inputs
%%%%%%%%%%%%%%%%%%%%%%%%%%%%%%%%%%%%%%%%%%%%%%%%%%%%%%%%%%%%%%%%%%%%%%%%%
% u (rad)       : current wrapped angle
% u_pre (rad)   : previous wrapped angle
% y_pre (rad)   : previous unwrapped angle

%%%%%%%%%%%%%%%%%%%%%%%%%%%%%%%%%%%%%%%%%%%%%%%%%%%%%%%%%%%%%%%%%%%%%%%%%
% Output
%%%%%%%%%%%%%%%%%%%%%%%%%%%%%%%%%%%%%%%%%%%%%%%%%%%%%%%%%%%%%%%%%%%%%%%%%
% y (rad)       : unwrapped angle
% u_next (rad)  : next wrapped angle

x = mod((u-hold)+pi, 2*pi) - pi;

y = y_pre + x;
hold = u;

end

== matlab function GNC2026/3 - Control/Default LQR Control (BLACK)/Calculate Error/MATLAB Function ==
  data: Rz_path input; Rz_error output; Rz_measured input
function Rz_error = SmoothAngularDifference(Rz_path, Rz_measured)

    Rz_error = mod(Rz_measured-Rz_path+pi, 2*pi)-pi;


end

== matlab function GNC2026/2 - Guidance/Custom PPL (RED)/Unwrap1/Unwrap/MATLAB Function ==
  data: u input; y output; u_pre input; y_pre input; u_next output
function [y, u_next] = fcn(u, u_pre, y_pre)

% Nimish Dhawan 2025
% Carleton University

%%%%%%%%%%%%%%%%%%%%%%%%%%%%%%%%%%%%%%%%%%%%%%%%%%%%%%%%%%%%%%%%%%%%%%%%%
% Inputs
%%%%%%%%%%%%%%%%%%%%%%%%%%%%%%%%%%%%%%%%%%%%%%%%%%%%%%%%%%%%%%%%%%%%%%%%%
% u (rad)       : current wrapped angle
% u_pre (rad)   : previous wrapped angle
% y_pre (rad)   : previous unwrapped angle

%%%%%%%%%%%%%%%%%%%%%%%%%%%%%%%%%%%%%%%%%%%%%%%%%%%%%%%%%%%%%%%%%%%%%%%%%
% Output
%%%%%%%%%%%%%%%%%%%%%%%%%%%%%%%%%%%%%%%%%%%%%%%%%%%%%%%%%%%%%%%%%%%%%%%%%
% y (rad)       : unwrapped angle
% u_next (rad)  : next wrapped angle

x = mod((u-u_pre)+pi, 2*pi) - pi;

y = y_pre + x;
u_next = u;

end

== matlab function GNC2026/2 - Guidance/Custom PPL (RED)/Unwrap1/Unwrap1/MATLAB Function ==
  data: u input; y output; y_pre input; init_states_BLACK parameter
function y  = fcn(u, y_pre, init_states_BLACK)

% Nimish Dhawan 2025
% Carleton University

persistent hold

if isempty(hold)
    hold = init_states_BLACK(3);
end

%%%%%%%%%%%%%%%%%%%%%%%%%%%%%%%%%%%%%%%%%%%%%%%%%%%%%%%%%%%%%%%%%%%%%%%%%
% Inputs
%%%%%%%%%%%%%%%%%%%%%%%%%%%%%%%%%%%%%%%%%%%%%%%%%%%%%%%%%%%%%%%%%%%%%%%%%
% u (rad)       : current wrapped angle
% u_pre (rad)   : previous wrapped angle
% y_pre (rad)   : previous unwrapped angle

%%%%%%%%%%%%%%%%%%%%%%%%%%%%%%%%%%%%%%%%%%%%%%%%%%%%%%%%%%%%%%%%%%%%%%%%%
% Output
%%%%%%%%%%%%%%%%%%%%%%%%%%%%%%%%%%%%%%%%%%%%%%%%%%%%%%%%%%%%%%%%%%%%%%%%%
% y (rad)       : unwrapped angle
% u_next (rad)  : next wrapped angle

x = mod((u-hold)+pi, 2*pi) - pi;

y = y_pre + x;
hold = u;

end

== matlab function GNC2026/Thruster Control Code/Change RED Behavior/Calculate Duty Cycle/MATLAB Function8 ==
  data: ThrustPer_Final output; ThrustPer input; PWMFreq parameter
function ThrustPer_Final  = ThrusterSat(ThrustPer, PWMFreq)

    ValveTime       = 0.007;
    TControl        = 1/PWMFreq;

    ThrustPer_Final = zeros(8,1);
    
    if max(ThrustPer) > 1
        ThrustPer_Sat = ThrustPer/max(ThrustPer);
    else
        ThrustPer_Sat = ThrustPer;
    end
    
    for i = 1:8
        if ThrustPer_Sat(i) > ValveTime/TControl 
            ThrustPer_Final(i) = ThrustPer_Sat(i);
        else
            ThrustPer_Final(i) = 0;
        end
    end


end

== matlab function GNC2026/Navigation Filter/If Action Subsystem/MEKF/Camera to Inertial Frame ==
  data: r_C_I input; r_T_I output; r_REL_C input
function r_T_I  = CIB(r_C_I, r_REL_C)
l_cam_x    = 0.125; %m, offset in x from origin of Red, left camera
l_cam_y    = 0.03; %m, offset in y from origin of Red, left camera
LAR_x      = 0.145; %m

r_REL_C(1:2) = r_REL_C(1:2) + [l_cam_x; l_cam_y];
th_C         = r_C_I(3);
th_REL       = r_REL_C(3);
th_T         = th_C+th_REL;

C_IC         = [cos(th_C) -sin(th_C); sin(th_C) cos(th_C)]; % Chaser to inertial ref frame rotation matrix
C_IT         = [cos(th_T) -sin(th_T); sin(th_T) cos(th_T)]; % Target to inertial ref frame rotation matrix
xy_T_I       = r_C_I(1:2) + C_IC*r_REL_C(1:2);

r_T_I        = [xy_T_I-C_IT*[LAR_x;0]; th_T];
end

== matlab function GNC2026/Simulate Plant Dynamics/RED and ARM Dynamics/RED + ARM/Dynamics Model ==
  data: q_dot output; x input; InertiaS input; CoriolisS input; u input; Gamma1_sh parameter; Gamma2_sh parameter; Gamma3_sh parameter; Gamma5_sh parameter; Gamma4_sh parameter; Gamma6_sh parameter; Gamma1_el parameter; Gamma2_el parameter; Gamma3_el parameter; Gamma5_el parameter; Gamma4_el parameter; Gamma6_el parameter; Gamma1_wr parameter; Gamma2_wr parameter; Gamma3_wr parameter; Gamma5_wr parameter; Gamma4_wr parameter; Gamma6_wr parameter; q_ddot output
function [q_dot, q_ddot]  = DynamicsModel(x, InertiaS, CoriolisS, u,...
    Gamma1_sh, Gamma2_sh, Gamma3_sh, Gamma5_sh, Gamma4_sh, Gamma6_sh,...
    Gamma1_el, Gamma2_el, Gamma3_el, Gamma5_el, Gamma4_el, Gamma6_el,...
    Gamma1_wr, Gamma2_wr, Gamma3_wr, Gamma5_wr, Gamma4_wr, Gamma6_wr)


    fqdot1 = Gamma1_sh*(tanh(Gamma2_sh*x(10)) - tanh(Gamma3_sh*x(10))) + Gamma4_sh*tanh(Gamma5_sh*x(10)) + Gamma6_sh*x(10);

    fqdot2 = Gamma1_el*(tanh(Gamma2_el*x(11)) - tanh(Gamma3_el*x(11))) + Gamma4_el*tanh(Gamma5_el*x(11)) + Gamma6_el*x(11);

    fqdot3 = Gamma1_wr*(tanh(Gamma2_wr*x(12)) - tanh(Gamma3_wr*x(12))) + Gamma4_wr*tanh(Gamma5_wr*x(12)) + Gamma6_wr*x(12);
    
    q_dot  = x(7:12);
    q_ddot = pinv(InertiaS)*(u - CoriolisS*x(7:12) - [0;0;0;fqdot1;fqdot2;fqdot3]);
    
end

== matlab function GNC2026/Navigation Filter/If Action Subsystem/MEKF/MEKF ==
  data: black_cv_pose input; pose output; velocity output; baseRate parameter; CVrate parameter; confidence output
% Ally Colla
% Chris El-Asmar
% DOT 2026 2D MEKF

function [pose, velocity, confidence] = MEKF(black_cv_pose, baseRate, CVrate)

persistent converge

if isempty(converge)
    converge = 0;
end

% process noise covariance for propogation
Qx = 1e-8;
Qy = 1e-8;
Qvx = 1e-8;
Qvy = 1e-8;
Qdtheta = 1e-8;
Qomega = 1e-8;

Qc = diag([Qx, Qy, Qvx, Qvy, Qdtheta, Qomega]);

% measurement noise covariance for measurement update
Rx = 5e-3;
Ry = 5e-3;
Rtheta = 5e-3;

R = diag([Rx, Ry, Rtheta]);

% filter initial conditions and memory
persistent x q P run theta_prev theta_cont

if isempty(run) % check if MEKF has run

    x = zeros(5,1); % x = state vector without theta [x, y, vx, vy, omega]
    q = 1 + 0i; % set angle to zero, store theta to update seperately 
    P = diag([1 1 0.05 0.05 0.1 0.05]); % initial uncertainties based off the spike magnitudes
    theta_prev = 0;
    theta_cont = 0;
    run = true;
end

% PROPOGATION

% positions
x(1) = x(1) + x(3)*baseRate; % updates x position, xnew = x+vx*dt
x(2) = x(2) + x(4)*baseRate; % updates y position, ynew = y+vy*dt

% attitude 
q = q*exp(1i*x(5)*baseRate); % quaternion equation
q = q/abs(q); % normalize q

% setting up state transition matrix 
phi = eye(6);
phi(1,3) = baseRate; 
phi(2,4) = baseRate; 
phi(5,6) = baseRate;

% calculating covariance of state estimation error
P = phi*P*phi.'+ Qc*baseRate;

% MEASUREMENT UPDATE AND MAHALANOBIS GATING

yk = black_cv_pose(:); % measurement vector from equation 23

theta = angle(q); % phase angle 
yk_pred = [x(1); x(2); theta]; % filter predicted state

% innovation equation
ik = yk - yk_pred;
ik(3) = atan2(sin(ik(3)), cos(ik(3))); % wrapping theta
if norm(ik) < 0.05
    converge = 1;
end
confidence = converge;

H = zeros(3,6);
H(1,1) = 1; % x
H(2,2) = 1; % y 
H(3,5) = 1; % theta

% innovation covariance
E_ik = H*P*H.'+ R; % linearized approximation, equation 26

% mahalanobis gate
d2 = ik.'/E_ik * ik; % calculate d(k)^2, equation 25
if d2 <= 7.815 % 95 percent confidence

    K = P*H.'/E_ik; % kalman gain
    delta_x = K * ik; % error state estimate

    x(1:4) = x(1:4) + delta_x(1:4); % additive update for other states 
    
    delta_theta = delta_x(5);
    q = q*exp(1i*delta_theta); % quaternion update for theta
    q = q/abs(q); % normalize 
    
    x(5) = x(5) + delta_x(6); % updating omega additively
    
    I = eye(6);
    % joseph form equation
    P = (I-K*H)*P*(I-K*H).'+K*R*K.';
end

% keeping theta continuous
theta = angle(q);
dtheta = atan2(sin(theta - theta_prev), cos(theta - theta_prev));
theta_cont = theta_cont + dtheta;
theta_prev = theta;

% extract position and velocities from state vector
pose = [x(1); x(2); theta_cont];
velocity = [x(3); x(4); x(5)];
end

% newMeas = measurement_flag(baseRate, CVrate);
% 
% x_plus = x_minus + delta_x;
% x_minus = x;
% P_minus = P;
% q_minus = q;
% 
% if isValid == 1 && newMeas == 1 
%     x_est = x_plus;
%     P_est = P_plus;
% else
%     x_est = x_minus;
%     P_est = P_minus;
% end
% 
% end

% :)

%%
function [flag] = measurement_flag(baseRate, CVrate)

persistent k
if isempty(k)
    k = 0;
end

flag = 0;

if mod(k,CVrate/baseRate) == 0      
    flag = 1;     % new measurement available
end

k = k + 1;

end

== matlab function GNC2026/Navigation Filter/If Action Subsystem/MEKF/Unwrap/Unwrap/MATLAB Function ==
  data: u input; y output; u_pre input; y_pre input; u_next output
function [y, u_next] = fcn(u, u_pre, y_pre)

% Nimish Dhawan 2025
% Carleton University

%%%%%%%%%%%%%%%%%%%%%%%%%%%%%%%%%%%%%%%%%%%%%%%%%%%%%%%%%%%%%%%%%%%%%%%%%
% Inputs
%%%%%%%%%%%%%%%%%%%%%%%%%%%%%%%%%%%%%%%%%%%%%%%%%%%%%%%%%%%%%%%%%%%%%%%%%
% u (rad)       : current wrapped angle
% u_pre (rad)   : previous wrapped angle
% y_pre (rad)   : previous unwrapped angle

%%%%%%%%%%%%%%%%%%%%%%%%%%%%%%%%%%%%%%%%%%%%%%%%%%%%%%%%%%%%%%%%%%%%%%%%%
% Output
%%%%%%%%%%%%%%%%%%%%%%%%%%%%%%%%%%%%%%%%%%%%%%%%%%%%%%%%%%%%%%%%%%%%%%%%%
% y (rad)       : unwrapped angle
% u_next (rad)  : next wrapped angle

x = mod((u-u_pre)+pi, 2*pi) - pi;

y = y_pre + x;
u_next = u;

end

== matlab function GNC2026/3 - Control/Default PD Control (RED)/Calculate Error/MATLAB Function ==
  data: Rz_path input; Rz_error output; Rz_measured input
function Rz_error = SmoothAngularDifference(Rz_path, Rz_measured)

    Rz_error = mod(Rz_measured-Rz_path+pi, 2*pi)-pi;


end

== matlab function GNC2026/Navigation Filter/If Action Subsystem/MEKF/Unwrap/Unwrap1/MATLAB Function ==
  data: u input; y output; y_pre input; init_states_BLACK parameter
function y  = fcn(u, y_pre, init_states_BLACK)

% Nimish Dhawan 2025
% Carleton University

persistent hold

if isempty(hold)
    hold = init_states_BLACK(3);
end

%%%%%%%%%%%%%%%%%%%%%%%%%%%%%%%%%%%%%%%%%%%%%%%%%%%%%%%%%%%%%%%%%%%%%%%%%
% Inputs
%%%%%%%%%%%%%%%%%%%%%%%%%%%%%%%%%%%%%%%%%%%%%%%%%%%%%%%%%%%%%%%%%%%%%%%%%
% u (rad)       : current wrapped angle
% u_pre (rad)   : previous wrapped angle
% y_pre (rad)   : previous unwrapped angle

%%%%%%%%%%%%%%%%%%%%%%%%%%%%%%%%%%%%%%%%%%%%%%%%%%%%%%%%%%%%%%%%%%%%%%%%%
% Output
%%%%%%%%%%%%%%%%%%%%%%%%%%%%%%%%%%%%%%%%%%%%%%%%%%%%%%%%%%%%%%%%%%%%%%%%%
% y (rad)       : unwrapped angle
% u_next (rad)  : next wrapped angle

x = mod((u-hold)+pi, 2*pi) - pi;

y = y_pre + x;
hold = u;

end

== matlab function GNC2026/3 - Control/Default PD Control (BLACK)/Calculate Error/MATLAB Function ==
  data: Rz_path input; Rz_error output; Rz_measured input
function Rz_error = SmoothAngularDifference(Rz_path, Rz_measured)

    Rz_error = mod(Rz_measured-Rz_path+pi, 2*pi)-pi;


end
